simulink model "Project6"  (R2014a)
settings: Solver=ode45  StartTime=0.0  StopTime=10.0  RelTol=1e-3
undefined symbols (not defined in the file): Kd, Ki, Kp
settings Model: Creator=DZR3QN  LastModifiedBy=DZR3QN

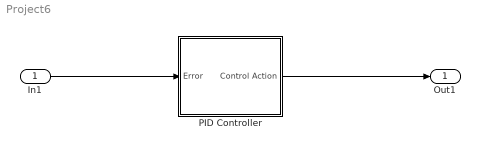
== system Project6 ==
  In1 : Inport
  PID Controller : Subsystem
  Out1 : Outport
  wires:
  In1/1 -> PID Controller/1(Error)
  PID Controller/1("Control Action ") -> Out1/1

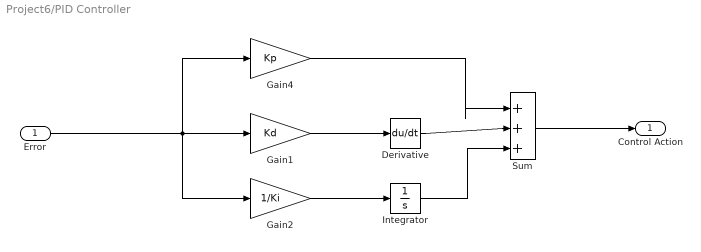
== system Project6/PID Controller ==
  Error : Inport
  Derivative : Derivative
  Gain1 : Gain  Gain=Kd
  Gain2 : Gain  Gain=1/Ki
  Gain4 : Gain  Gain=Kp
  Integrator : Integrator
  Sum : Sum  Inputs=|+++
  "Control Action " : Outport
  wires:
  Sum/1 -> "Control Action "/1
  Derivative/1 -> Sum/2
  Gain4/1 -> Sum/1
  Error/1 -> Gain2/1, Gain4/1, Gain1/1
  Gain1/1 -> Derivative/1
  Gain2/1 -> Integrator/1
  Integrator/1 -> Sum/3
